simulink model "v_f_control"  (R2014b)
settings: Solver=ode23tb  StartTime=0.0  StopTime=10.0  MaxStep=1e-4  RelTol=1e-3
libraries: powerlib x5, simulink x2
settings Model: Creator=Amr Saleh  LastModifiedBy=Amr Saleh

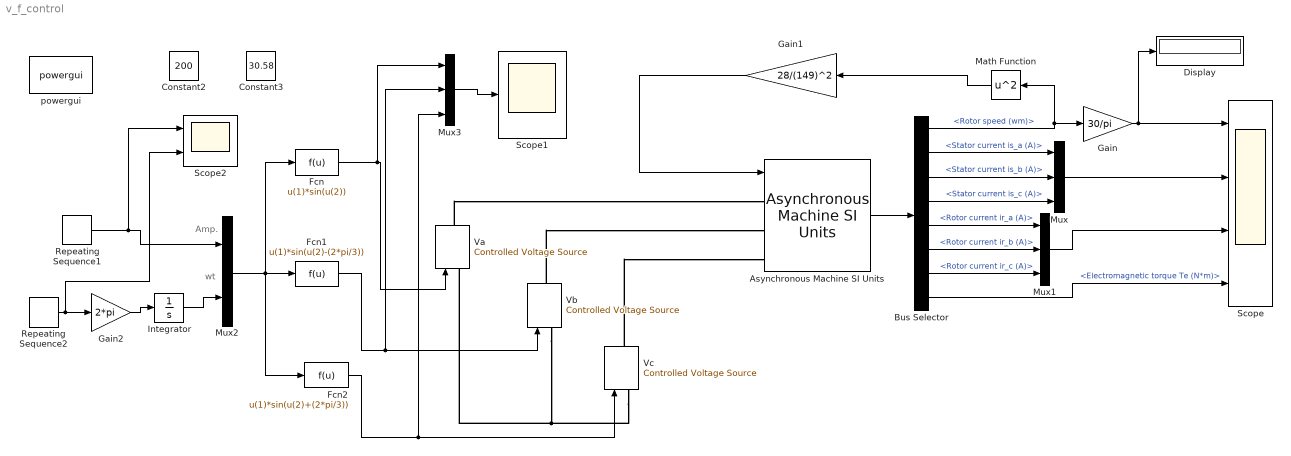
== system v_f_control ==
  note: wt
  note: Amp.
  Asynchronous Machine SI Units : powerlib/Machines/Asynchronous Machine SI Units  PresetModel="15:  5.4 HP (4KW)   400 V  50Hz 1430 RPM"  MechanicalLoad=Torque Tm  ShowDetailedParameters=on  RotorType=Squirrel-cage  ReferenceFrame=Rotor  Units=SI  MeasurementBus=off  NominalParameters=[4000 400 50]  Stator=[1.405 0.005839]  Rotor=[1.395 0.005839]  Cage1=[ 0.022 0.226/377]  Cage2=[ 0.022 0.226/377]  Lm=0.1722  Mechanical=[0.0131 0.002985 2]  PolePairs=2  InitialConditions=[1 0 0 0 0 0 0 0]  SimulateSaturation=off  Saturation=[14.03593122, 27.81365428, 53.79336849, 72.68890987, 97.98006896, 148.6815601, 215.7428561, 302.9841135, 420.4778367 ; 230, 322, 414, 460, 506, 552, 598, 644, 690]  LoadFlowParameters=1492000  TsPowergui=0  TsBlock=-1  IterativeModel=Trapezoidal non iterative  Pmec=0
  Bus Selector : BusSelector  OutputSignals=Mechanical.Rotor speed (wm),Stator measurements.Stator current is_a (A),Stator measurements.Stator current is_b (A),Stator measurements.Stator current is_c (A),Rotor measurements.Rotor current ir_a (A),Rotor measurements.Rotor current ir_b (A),Rotor measurements.Rotor current ir_c (A),Mechanical.Electromagnetic torque Te (N*m)
  Constant2 : Constant  Value=200
  Constant3 : Constant  Value=30.58
  Display : Display
  Fcn : Fcn  Expr=u(1)*sin(u(2))
  Fcn1 : Fcn  Expr=u(1)*sin(u(2)-(2*pi/3))
  Fcn2 : Fcn  Expr=u(1)*sin(u(2)+(2*pi/3))
  Gain : Gain  Gain=30/pi
  Gain1 : Gain  Gain=28/(149)^2
  Gain2 : Gain  Gain=2*pi
  Integrator : Integrator
  Math Function : Math  Operator=square  SaturateOnIntegerOverflow=on
  Mux : Mux  Inputs=3
  Mux1 : Mux  Inputs=3
  Mux2 : Mux  Inputs=2
  Mux3 : Mux  Inputs=3
  Repeating Sequence1 : simulink/Sources/Repeating Sequence  rep_seq_t=[0 0.2 10]  rep_seq_y=[0 327 327]
  Repeating Sequence2 : simulink/Sources/Repeating Sequence  rep_seq_t=[0 0.2 10]  rep_seq_y=[0 50 50]
  Scope : Scope  NumInputPorts=4
      settings: YMin=-5~-5~-5~-5  YMax=5~5~5~5
  Scope1 : Scope
  Scope2 : Scope  NumInputPorts=2
      settings: YMin=-5~-5  YMax=5~5  SaveName=ScopeData2
  Va : powerlib/Electrical Sources/Controlled Voltage Source  Initialize=on  Source_Type=AC  Amplitude=0  Phase=0  Frequency=0  Measurements=None
  Vb : powerlib/Electrical Sources/Controlled Voltage Source  Initialize=on  Source_Type=AC  Amplitude=0  Phase=0  Frequency=0  Measurements=None
  Vc : powerlib/Electrical Sources/Controlled Voltage Source  Initialize=on  Source_Type=AC  Amplitude=0  Phase=0  Frequency=0  Measurements=None
  powergui : powerlib/powergui  Priority=1  SimulationMode=Continuous  SolverType=Tustin/Backward Euler (TBE)  SampleTime=50e-6  frequency=60  SPID=off  DisableSnubberDevices=off  DisableRonSwitches=off  DisableVfSwitches=off  SwTol=0  DisplayEquations=off  Interpol=off  methode=off  Ts=100  frequencyindice=50  Pbase=100e6  ErrMax=1e-4  Iterations=50  UnitsV=kV  UnitsW=MW  FunctionMessages=off  echomessages=off  HookPort=off  EnableUseOfTLC=off  x0status=blocks  RestoreLinks=warning  ResistiveCurrentMeasurement=off  Frange=[0:2:500]  Ylog=off  Xlog=on  ShowGrid=off  save=off  variable=ZData  structure=0  ZoomFFT=off  StartTime=0.0  cycles=1  DisplayStyle=1  fundamental=60  FreqAxis=off  MaxFrequency=1000  frequencyindicesteady=1  RmsSteady=1  display=off
  wires:
  Gain1/1 -> Asynchronous Machine SI Units/1
  Asynchronous Machine SI Units/1 -> Bus Selector/1
  Bus Selector/2 -> Mux/1  "<Stator current is_a (A)>"
  Bus Selector/3 -> Mux/2  "<Stator current is_b (A)>"
  Bus Selector/4 -> Mux/3  "<Stator current is_c (A)>"
  Bus Selector/6 -> Mux1/2  "<Rotor current ir_b (A)>"
  Bus Selector/7 -> Mux1/3  "<Rotor current ir_c (A)>"
  Bus Selector/5 -> Mux1/1  "<Rotor current ir_a (A)>"
  Bus Selector/1 -> Math Function/1, Gain/1  "<Rotor speed (wm)>"
  Bus Selector/8 -> Scope/4  "<Electromagnetic torque Te (N*m)>"
  Mux/1 -> Scope/2
  Mux1/1 -> Scope/3
  Gain/1 -> Display/1, Scope/1
  Math Function/1 -> Gain1/1
  Mux2/1 -> Fcn/1, Fcn1/1, Fcn2/1
  Fcn/1 -> Mux3/1, Va/1
  Fcn1/1 -> Mux3/2, Vb/1
  Fcn2/1 -> Mux3/3, Vc/1
  Repeating Sequence1/1 -> Scope2/1, Mux2/1
  Repeating Sequence2/1 -> Scope2/2, Gain2/1
  Gain2/1 -> Integrator/1
  Integrator/1 -> Mux2/2
  Mux3/1 -> Scope1/1
  connections:
  Va/RConn1 -- Asynchronous Machine SI Units/LConn1
  Vb/RConn1 -- Asynchronous Machine SI Units/LConn2
  Vc/RConn1 -- Asynchronous Machine SI Units/LConn3
  Vc/LConn1 -- Vb/LConn1 -- Va/LConn1
